simulink model "SAFE"  (R2014b)
settings: Solver=ode4  StartTime=0  StopTime=15000  FixedStep=ConfParam.confOrbit.dt  RelTol=1e-3
undefined symbols (not defined in the file): ConfParam
libraries: BdotController x1, Date x1, KepOrbit x1, DipoleField x1, SunEphemeris_MathWorks x1, MTB x1, Magnetometer x1, AeroTorqueA x1, GravGradTorque x1, MagnTorque x1, SunTorqueA x1, SatDyn x1
settings Model: Creator=Hp  LastModifiedBy=Hp
settings DataIOCC: SaveTime=off
settings DebuggingCC: MultiTaskRateTransMsg=warning

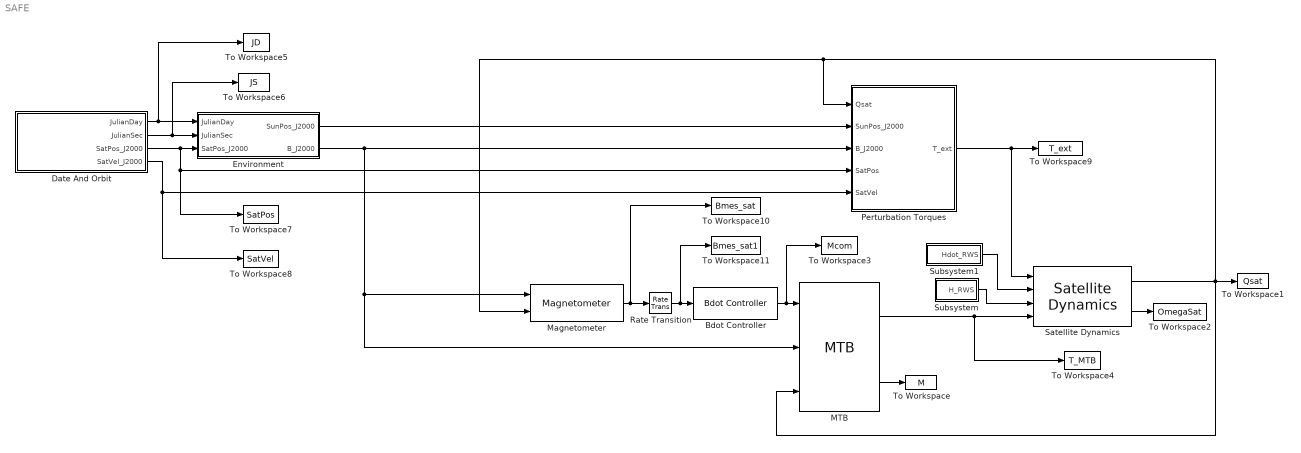
== system SAFE ==
  Bdot Controller : BdotController/Bdot Controller
  Date And Orbit : Subsystem
  Environment : Subsystem
  MTB : MTB/MTB
  Magnetometer : Magnetometer/Magnetometer
  Perturbation Torques : Subsystem
  Rate Transition : RateTransition  X0=[0;0;0]  OutPortSampleTime=1/ConfParam.confES.frequency
  Satellite Dynamics : SatDyn/Satellite Dynamics
  Subsystem : Subsystem
  Subsystem1 : Subsystem
  To Workspace : ToWorkspace  VariableName=M  SaveFormat=Timeseries  SampleTime=-1
  To Workspace1 : ToWorkspace  VariableName=Qsat  SaveFormat=Timeseries  SampleTime=-1
  To Workspace10 : ToWorkspace  VariableName=Bmes_sat  SaveFormat=Timeseries  SampleTime=-1
  To Workspace11 : ToWorkspace  VariableName=Bmes_sat1  SaveFormat=Timeseries  SampleTime=-1
  To Workspace2 : ToWorkspace  VariableName=OmegaSat  SaveFormat=Timeseries  SampleTime=-1
  To Workspace3 : ToWorkspace  VariableName=Mcom  SaveFormat=Timeseries  SampleTime=-1
  To Workspace4 : ToWorkspace  VariableName=T_MTB  SaveFormat=Timeseries  SampleTime=-1
  To Workspace5 : ToWorkspace  VariableName=JD  SaveFormat=Timeseries  SampleTime=-1
  To Workspace6 : ToWorkspace  VariableName=JS  SaveFormat=Timeseries  SampleTime=-1
  To Workspace7 : ToWorkspace  VariableName=SatPos  SaveFormat=Timeseries  SampleTime=-1
  To Workspace8 : ToWorkspace  VariableName=SatVel  SaveFormat=Timeseries  SampleTime=-1
  To Workspace9 : ToWorkspace  VariableName=T_ext  SaveFormat=Timeseries  SampleTime=-1
  wires:
  Environment/2(B_J2000) -> Perturbation Torques/3(B_J2000), Magnetometer/1, MTB/2
  Environment/1(SunPos_J2000) -> Perturbation Torques/2(SunPos_J2000)
  Date And Orbit/3(SatPos_J2000) -> To Workspace7/1, Perturbation Torques/4(SatPos), Environment/3(SatPos_J2000)
  Date And Orbit/4(SatVel_J2000) -> To Workspace8/1, Perturbation Torques/5(SatVel)
  Date And Orbit/1(JulianDay) -> To Workspace5/1, Environment/1(JulianDay)
  Date And Orbit/2(JulianSec) -> To Workspace6/1, Environment/2(JulianSec)
  MTB/1 -> To Workspace4/1, Satellite Dynamics/4
  Perturbation Torques/1(T_ext) -> Satellite Dynamics/1, To Workspace9/1
  Satellite Dynamics/1 -> To Workspace1/1, Perturbation Torques/1(Qsat), Magnetometer/2, MTB/3
  Subsystem1/1(Hdot_RWS) -> Satellite Dynamics/2
  Subsystem/1(H_RWS) -> Satellite Dynamics/3
  Magnetometer/1 -> Rate Transition/1, To Workspace10/1
  Bdot Controller/1 -> To Workspace3/1, MTB/1
  Rate Transition/1 -> To Workspace11/1, Bdot Controller/1
  MTB/2 -> To Workspace/1
  Satellite Dynamics/2 -> To Workspace2/1

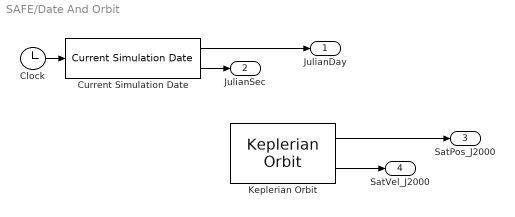
== system SAFE/Date And Orbit ==
  Clock : Clock
      settings: Decimation=1/ConfParam.confOrbit.dt
  Current Simulation Date : Date/Current Simulation Date
  Keplerian Orbit : KepOrbit/Keplerian Orbit
  JulianDay : Outport
  JulianSec : Outport  Port=2
  SatPos_J2000 : Outport  Port=3
  SatVel_J2000 : Outport  Port=4
  wires:
  Keplerian Orbit/2 -> SatVel_J2000/1
  Clock/1 -> Current Simulation Date/1
  Current Simulation Date/1 -> JulianDay/1
  Keplerian Orbit/1 -> SatPos_J2000/1
  Current Simulation Date/2 -> JulianSec/1

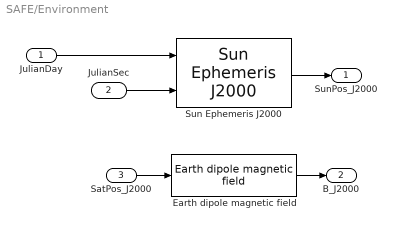
== system SAFE/Environment ==
  JulianDay : Inport
  JulianSec : Inport  Port=2
  SatPos_J2000 : Inport  Port=3
  Earth dipole magnetic field : DipoleField/Earth dipole magnetic field
  Sun Ephemeris J2000 : SunEphemeris_MathWorks/Sun Ephemeris J2000
  SunPos_J2000 : Outport
  B_J2000 : Outport  Port=2
  wires:
  Earth dipole magnetic field/1 -> B_J2000/1
  Sun Ephemeris J2000/1 -> SunPos_J2000/1
  JulianSec/1 -> Sun Ephemeris J2000/2
  SatPos_J2000/1 -> Earth dipole magnetic field/1
  JulianDay/1 -> Sun Ephemeris J2000/1

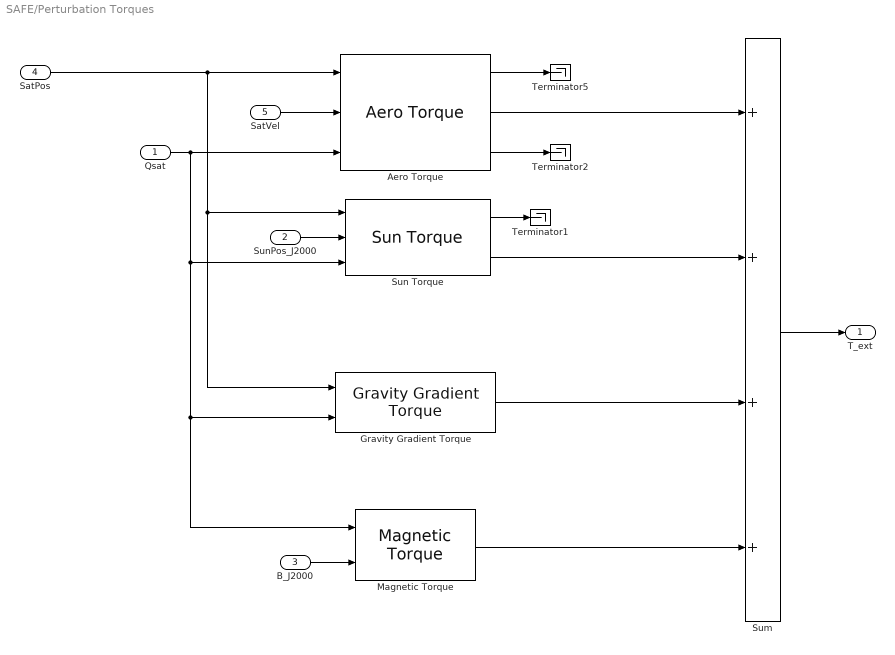
== system SAFE/Perturbation Torques ==
  Qsat : Inport
  SunPos_J2000 : Inport  Port=2
  B_J2000 : Inport  Port=3
  SatPos : Inport  Port=4
  SatVel : Inport  Port=5
  Aero Torque : AeroTorqueA/Aero Torque
  Gravity Gradient Torque : GravGradTorque/Gravity Gradient Torque
  Magnetic Torque : MagnTorque/Magnetic Torque
  Sum : Sum  Inputs=++++
  Sun Torque : SunTorqueA/Sun Torque
  Terminator1 : Terminator
  Terminator2 : Terminator
  Terminator5 : Terminator
  T_ext : Outport
  wires:
  SunPos_J2000/1 -> Sun Torque/2
  SatVel/1 -> Aero Torque/2
  Qsat/1 -> Aero Torque/3, Gravity Gradient Torque/2, Magnetic Torque/1, Sun Torque/3
  Gravity Gradient Torque/1 -> Sum/3
  B_J2000/1 -> Magnetic Torque/2
  Sum/1 -> T_ext/1
  Magnetic Torque/1 -> Sum/4
  Aero Torque/1 -> Terminator5/1
  SatPos/1 -> Aero Torque/1, Gravity Gradient Torque/1, Sun Torque/1
  Aero Torque/3 -> Terminator2/1
  Aero Torque/2 -> Sum/1
  Sun Torque/1 -> Terminator1/1
  Sun Torque/2 -> Sum/2

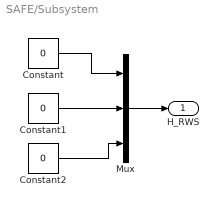
== system SAFE/Subsystem ==
  Constant : Constant  Value=0
  Constant1 : Constant  Value=0
  Constant2 : Constant  Value=0
  Mux : Mux  Inputs=3
  H_RWS : Outport
  wires:
  Mux/1 -> H_RWS/1
  Constant1/1 -> Mux/2
  Constant/1 -> Mux/1
  Constant2/1 -> Mux/3

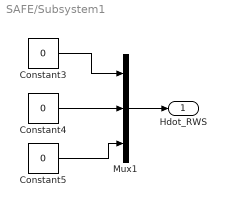
== system SAFE/Subsystem1 ==
  Constant3 : Constant  Value=0
  Constant4 : Constant  Value=0
  Constant5 : Constant  Value=0
  Mux1 : Mux  Inputs=3
  Hdot_RWS : Outport
  wires:
  Constant5/1 -> Mux1/3
  Mux1/1 -> Hdot_RWS/1
  Constant3/1 -> Mux1/1
  Constant4/1 -> Mux1/2
